simulink model "Observador_Estados_continuo_plantilla"  (R2016a)
settings: Solver=VariableStepAuto  StartTime=0.0  StopTime=inf  RelTol=1e-3
values from neighbouring files (symbols this model uses):
  b = 1    [Repaso_represent_var_est_func_trans.m]
  h = place(A',C',Po)'    [Control_sist_no_lineal_punto_operacion.m]    (also in Observador_Estados.m = h'; Observador_Estados_codigo_matlab.m = h')
  kp = k(1:1,1:2)    [Control_sist_no_lineal_punto_operacion.m]    (also in Observador_Estados_codigo_matlab.m = k(:,1:2))
undefined symbols (not defined in the file or in its folder): a, c, ks, National_Instruments, PCI
libraries: sldrtlib x2, simulink x1
settings Model: Creator=Daniel  LastModifiedBy=daniel.tobon

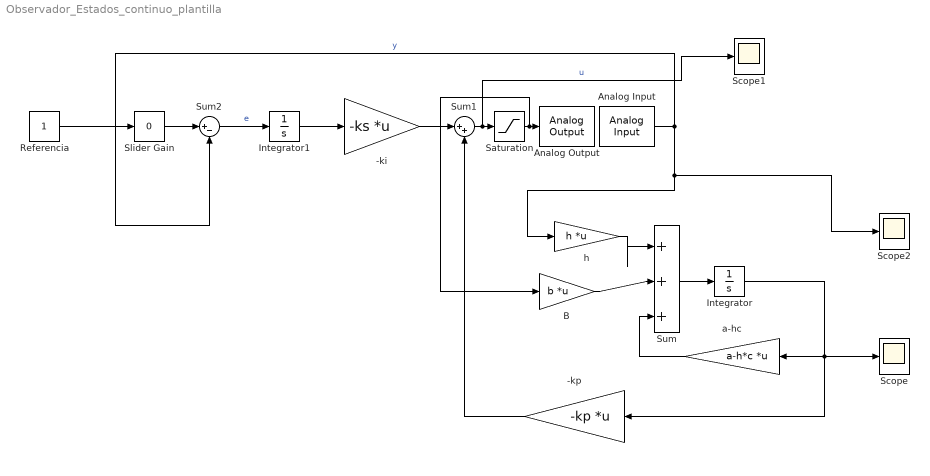
== system Observador_Estados_continuo_plantilla ==
  -ki : Gain  Gain=-ks  Multiplication=Matrix(K*u) (u vector)
  -kp : Gain  Gain=-kp  Multiplication=Matrix(K*u) (u vector)
  Analog Input : sldrtlib/Analog Input  SampleTime=0.1  MaxMissedTicks=10  ShowMissedTicks=off  YieldWhenWaiting=off  DrvName=National_Instruments/PCI-6221  DrvAddress=4294967295  DrvOptions=[1 0 0 0 0]  Channels=4  RangeMode=1  VoltRange=2  DataType=1
      settings: AttributesFormatString=National Instruments\nPCI-6221 [auto]
  Analog Output : sldrtlib/Analog Output  SampleTime=0.1  MaxMissedTicks=10  ShowMissedTicks=off  YieldWhenWaiting=off  DrvName=National_Instruments/PCI-6221  DrvAddress=4294967295  DrvOptions=[1 0 0 0 0]  Channels=1  RangeMode=1  VoltRange=1  InitialValue=[]  FinalValue=[]
      settings: AttributesFormatString=National Instruments\nPCI-6221 [auto]
  B : Gain  Gain=b  Multiplication=Matrix(K*u) (u vector)
  Integrator : Integrator
  Integrator1 : Integrator
  Referencia : Constant
  Saturation : Saturate  UpperLimit=6  LowerLimit=0
  Scope : Scope
  Scope1 : Scope
  Scope2 : Scope
  Slider Gain : simulink/Math Operations/Slider Gain  low=0  gain=0  high=5
  Sum : Sum  Inputs=|+++
  Sum1 : Sum  Inputs=|++
  Sum2 : Sum  Inputs=|+-
  a-hc : Gain  Gain=a-h*c  Multiplication=Matrix(K*u) (u vector)
  h : Gain  Gain=h  Multiplication=Matrix(K*u) (u vector)
  wires:
  Sum/1 -> Integrator/1
  a-hc/1 -> Sum/3
  B/1 -> Sum/2
  h/1 -> Sum/1
  Analog Input/1 -> Scope2/1, h/1, Sum2/2  "y"
  Sum1/1 -> Scope1/1, Saturation/1  "u"
  Integrator1/1 -> -ki/1
  Sum2/1 -> Integrator1/1  "e"
  Referencia/1 -> Slider Gain/1
  -ki/1 -> Sum1/1
  Integrator/1 -> Scope/1, -kp/1, a-hc/1
  -kp/1 -> Sum1/2
  Saturation/1 -> B/1, Analog Output/1
  Slider Gain/1 -> Sum2/1
